simulink model "All_Controllers"  (R2019b)
settings: Solver=VariableStepAuto  StartTime=0.0  StopTime=100  RelTol=1e-3
values from neighbouring files (symbols this model uses):
  A = data(1:1500, 1:3)    [ANN4.m]
  bike_params = [g h b a lambda m]    [All_ControllersScript.m]
  FinalValue = 1    [All_ControllersScript.m]
  Init_Angle = 0    [All_ControllersScript.m]
  lambda = deg2rad(90-24)    [All_ControllersScript.m]
  Noise = 1    [All_ControllersScript.m]
  PathData = length(SimulinkPath)-1    [All_ControllersScript.m]
  sys_dicretePID = c2d(steer_sys, Tsm, 'matched')    [All_ControllersScript.m]
  Ts = 0.01    [All_ControllersScript.m]
  TsD = 0.1    [All_ControllersScript.m]
  Tsm = Ts/6    (= 0.00166666666667)    [All_ControllersScript.m]
  v = 14/3.6    (= 3.88888888889)    [All_ControllersScript.m]
undefined symbols (not defined in the file or in its folder): B, C, D
libraries: simulink x9, simulink_extras x5, dspsrcs4 x1, dspsigops x1
settings Model: Creator=npn13003  LastModifiedBy=hampu
settings DataIOCC: ReturnWorkspaceOutputs=off
settings DebuggingCC: ArithmeticOperatorsInVariantConditions=warning
settings SFSimCC: SimUseLocalCustomCode=off  CustomCodeUndefinedFunction=UseInterfaceOnly
settings RTWCC: RTWUseLocalCustomCode=off

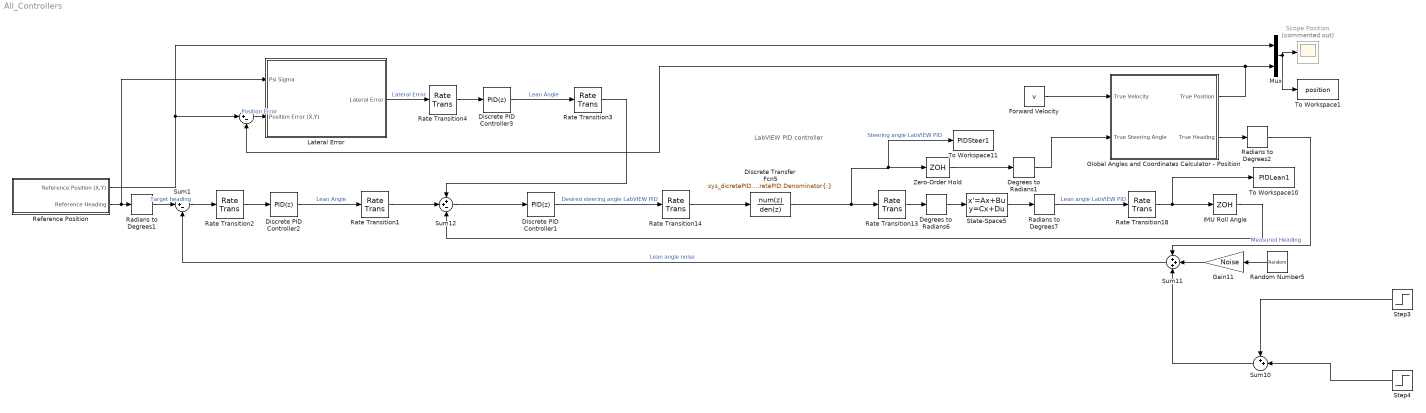
== system All_Controllers ==
  note: LabVIEW PID controller
  " " : Sum  Inputs=|+-
  Degrees to Radians1 : simulink_extras/Transformations/Degrees to Radians
  Degrees to Radians6 : simulink_extras/Transformations/Degrees to Radians
  Discrete Transfer Fcn5 : DiscreteTransferFcn  Numerator=sys_dicretePID.Numerator{:}  Denominator=sys_dicretePID.Denominator{:}
  Discrete PID Controller1 : simulink/Continuous/PID Controller  Controller=PID  Form=Ideal  TimeDomain=Discrete-time  SampleTime=Ts  IntegratorMethod=Trapezoidal  FilterMethod=Forward Euler  ControllerParametersSource=internal  P=3.418  I=1.327  D=0.0646  UseFilter=off  N=100  TunerSelectOption=Transfer Function Based (PID Tuner App)  InitialConditionSource=internal  InitialConditionForIntegrator=0  InitialConditionForFilter=0  DifferentiatorICPrevScaledInput=0  ExternalReset=none  TrackingMode=off  Kt=1  LimitOutput=off  UpperSaturationLimit=inf  LowerSaturationLimit=-inf  LinearizeAsGain=off  AntiWindupMode=none  Kb=1  POutMin=[]  POutMax=[]  IOutMin=[]  IOutMax=[]  DOutMin=[]  DOutMax=[]  NOutMin=[]  NOutMax=[]  SumOutMin=[]  SumOutMax=[]  SaturationOutMin=[]  SaturationOutMax=[]  PParamMin=[]  PParamMax=[]  IParamMin=[]  IParamMax=[]  DParamMin=[]  DParamMax=[]  NParamMin=[]  NParamMax=[]  KbParamMin=[]  KbParamMax=[]  KtParamMin=[]  KtParamMax=[]  KbOutMin=[]  KbOutMax=[]  KtOutMin=[]  KtOutMax=[]  IntegratorOutMin=[]  IntegratorOutMax=[]  FilterOutMin=[]  FilterOutMax=[]  SumI1OutMin=[]  SumI1OutMax=[]  SumI2OutMin=[]  SumI2OutMax=[]  SumI3OutMin=[]  SumI3OutMax=[]  SumI4OutMin=[]  SumI4OutMax=[]  SumDOutMin=[]  SumDOutMax=[]  DifferentiatorOutMin=[]  DifferentiatorOutMax=[]  FilterDiffOutCoefMin=[]  FilterDiffOutCoefMax=[]  ReciprocalOutMin=[]  ReciprocalOutMax=[]  SumDenOutMin=[]  SumDenOutMax=[]  SumNumOutMin=[]  SumNumOutMax=[]  DivideOutMin=[]  DivideOutMax=[]  IntegratorContinuousStateAttributes=''  IntegratorStateMustResolveToSignalObject=off  IntegratorRTWStateStorageClass=Auto  FilterContinuousStateAttributes=''  FilterStateMustResolveToSignalObject=off  FilterRTWStateStorageClass=Auto  ParallelPVariant=Passthrough  IdealPVariant=InternalParameters  IVariant=InternalParameters  DVariant=InternalParameters  IntegratorVariant=Discrete  SatVariant=Disabled  AWVariant=Passthrough  PCopyVariant=Disabled  TRVariant=Disabled  FdbkBlocksVariant=Forward  IdealPFdbkVariant=Disabled  SatFdbkVariant=Disabled  DerivativeFilterVariant=Differentiator  NVariant=Passthrough  NCopyVariant=Disabled_SignalSpec  FilterICVariant=InternalICsDifferentiator  IntegratorICVariant=InternalICs  ExternalResetVariant=Disabled  TRSumVariant=Passthrough  SumFdbkVariant=Disabled  SumVariant=Sum_PID
  Discrete PID Controller2 : simulink/Continuous/PID Controller  Controller=PID  Form=Ideal  TimeDomain=Discrete-time  SampleTime=TsD  IntegratorMethod=Trapezoidal  FilterMethod=Forward Euler  ControllerParametersSource=internal  P=-0.2  I=0  D=0  UseFilter=off  N=100  TunerSelectOption=Transfer Function Based (PID Tuner App)  InitialConditionSource=internal  InitialConditionForIntegrator=0  InitialConditionForFilter=0  DifferentiatorICPrevScaledInput=0  ExternalReset=none  TrackingMode=off  Kt=1  LimitOutput=off  UpperSaturationLimit=inf  LowerSaturationLimit=-inf  LinearizeAsGain=off  AntiWindupMode=none  Kb=1  POutMin=[]  POutMax=[]  IOutMin=[]  IOutMax=[]  DOutMin=[]  DOutMax=[]  NOutMin=[]  NOutMax=[]  SumOutMin=[]  SumOutMax=[]  SaturationOutMin=[]  SaturationOutMax=[]  PParamMin=[]  PParamMax=[]  IParamMin=[]  IParamMax=[]  DParamMin=[]  DParamMax=[]  NParamMin=[]  NParamMax=[]  KbParamMin=[]  KbParamMax=[]  KtParamMin=[]  KtParamMax=[]  KbOutMin=[]  KbOutMax=[]  KtOutMin=[]  KtOutMax=[]  IntegratorOutMin=[]  IntegratorOutMax=[]  FilterOutMin=[]  FilterOutMax=[]  SumI1OutMin=[]  SumI1OutMax=[]  SumI2OutMin=[]  SumI2OutMax=[]  SumI3OutMin=[]  SumI3OutMax=[]  SumI4OutMin=[]  SumI4OutMax=[]  SumDOutMin=[]  SumDOutMax=[]  DifferentiatorOutMin=[]  DifferentiatorOutMax=[]  FilterDiffOutCoefMin=[]  FilterDiffOutCoefMax=[]  ReciprocalOutMin=[]  ReciprocalOutMax=[]  SumDenOutMin=[]  SumDenOutMax=[]  SumNumOutMin=[]  SumNumOutMax=[]  DivideOutMin=[]  DivideOutMax=[]  IntegratorContinuousStateAttributes=''  IntegratorStateMustResolveToSignalObject=off  IntegratorRTWStateStorageClass=Auto  FilterContinuousStateAttributes=''  FilterStateMustResolveToSignalObject=off  FilterRTWStateStorageClass=Auto  ParallelPVariant=Passthrough  IdealPVariant=InternalParameters  IVariant=InternalParameters  DVariant=InternalParameters  IntegratorVariant=Discrete  SatVariant=Disabled  AWVariant=Passthrough  PCopyVariant=Disabled  TRVariant=Disabled  FdbkBlocksVariant=Forward  IdealPFdbkVariant=Disabled  SatFdbkVariant=Disabled  DerivativeFilterVariant=Differentiator  NVariant=Passthrough  NCopyVariant=Disabled_SignalSpec  FilterICVariant=InternalICsDifferentiator  IntegratorICVariant=InternalICs  ExternalResetVariant=Disabled  TRSumVariant=Passthrough  SumFdbkVariant=Disabled  SumVariant=Sum_PID
  Discrete PID Controller3 : simulink/Continuous/PID Controller  Controller=PID  Form=Ideal  TimeDomain=Discrete-time  SampleTime=TsD  IntegratorMethod=Trapezoidal  FilterMethod=Forward Euler  ControllerParametersSource=internal  P=-2  I=0  D=0  UseFilter=off  N=100  TunerSelectOption=Transfer Function Based (PID Tuner App)  InitialConditionSource=internal  InitialConditionForIntegrator=0  InitialConditionForFilter=0  DifferentiatorICPrevScaledInput=0  ExternalReset=none  TrackingMode=off  Kt=1  LimitOutput=off  UpperSaturationLimit=inf  LowerSaturationLimit=-inf  LinearizeAsGain=off  AntiWindupMode=none  Kb=1  POutMin=[]  POutMax=[]  IOutMin=[]  IOutMax=[]  DOutMin=[]  DOutMax=[]  NOutMin=[]  NOutMax=[]  SumOutMin=[]  SumOutMax=[]  SaturationOutMin=[]  SaturationOutMax=[]  PParamMin=[]  PParamMax=[]  IParamMin=[]  IParamMax=[]  DParamMin=[]  DParamMax=[]  NParamMin=[]  NParamMax=[]  KbParamMin=[]  KbParamMax=[]  KtParamMin=[]  KtParamMax=[]  KbOutMin=[]  KbOutMax=[]  KtOutMin=[]  KtOutMax=[]  IntegratorOutMin=[]  IntegratorOutMax=[]  FilterOutMin=[]  FilterOutMax=[]  SumI1OutMin=[]  SumI1OutMax=[]  SumI2OutMin=[]  SumI2OutMax=[]  SumI3OutMin=[]  SumI3OutMax=[]  SumI4OutMin=[]  SumI4OutMax=[]  SumDOutMin=[]  SumDOutMax=[]  DifferentiatorOutMin=[]  DifferentiatorOutMax=[]  FilterDiffOutCoefMin=[]  FilterDiffOutCoefMax=[]  ReciprocalOutMin=[]  ReciprocalOutMax=[]  SumDenOutMin=[]  SumDenOutMax=[]  SumNumOutMin=[]  SumNumOutMax=[]  DivideOutMin=[]  DivideOutMax=[]  IntegratorContinuousStateAttributes=''  IntegratorStateMustResolveToSignalObject=off  IntegratorRTWStateStorageClass=Auto  FilterContinuousStateAttributes=''  FilterStateMustResolveToSignalObject=off  FilterRTWStateStorageClass=Auto  ParallelPVariant=Passthrough  IdealPVariant=InternalParameters  IVariant=InternalParameters  DVariant=InternalParameters  IntegratorVariant=Discrete  SatVariant=Disabled  AWVariant=Passthrough  PCopyVariant=Disabled  TRVariant=Disabled  FdbkBlocksVariant=Forward  IdealPFdbkVariant=Disabled  SatFdbkVariant=Disabled  DerivativeFilterVariant=Differentiator  NVariant=Passthrough  NCopyVariant=Disabled_SignalSpec  FilterICVariant=InternalICsDifferentiator  IntegratorICVariant=InternalICs  ExternalResetVariant=Disabled  TRSumVariant=Passthrough  SumFdbkVariant=Disabled  SumVariant=Sum_PID
  Forward Velocity : Constant  Value=v
  Gain11 : Gain  Gain=Noise
  Global Angles and Coordinates Calculator - Position : Subsystem  SystemSampleTime=Ts
  IMU Roll Angle : ZeroOrderHold  SampleTime=Ts
  Lateral Error : Subsystem  SystemSampleTime=Ts
  Mux : Mux  Inputs=2
  Radians to Degrees1 : simulink_extras/Transformations/Radians to Degrees
  Radians to Degrees2 : simulink_extras/Transformations/Radians to Degrees
  Radians to Degrees7 : simulink_extras/Transformations/Radians to Degrees
  Random Number5 : RandomNumber  Variance=0.0001  SampleTime=Ts
  Rate Transition1 : RateTransition  OutPortSampleTime=Ts
  Rate Transition13 : RateTransition  OutPortSampleTime=0
  Rate Transition14 : RateTransition  OutPortSampleTime=Tsm
  Rate Transition18 : RateTransition  OutPortSampleTime=Ts
  Rate Transition2 : RateTransition  OutPortSampleTime=TsD
  Rate Transition3 : RateTransition  OutPortSampleTime=Ts
  Rate Transition4 : RateTransition  OutPortSampleTime=TsD
  Reference Position : Subsystem
  Scope Position : Scope  Commented=on
  State-Space5 : StateSpace  A=A  B=B  C=C  D=D  InitialCondition=[deg2rad(Init_Angle/C(1,1)) 0]
  Step3 : Step  Time=1.25  After=-FinalValue  SampleTime=Ts  VectorParams1D=off
  Step4 : Step  After=FinalValue  SampleTime=Ts  VectorParams1D=off
  Sum1 : Sum  Inputs=|+-
  Sum10 : Sum  Inputs=++|
  Sum11 : Sum  Inputs=+++
  Sum12 : Sum  Inputs=++-
  To Workspace1 : ToWorkspace  VariableName=position  SaveFormat=Timeseries  SampleTime=-1
  To Workspace10 : ToWorkspace  VariableName=PIDLean1  SampleTime=-1
  To Workspace11 : ToWorkspace  VariableName=PIDSteer1  SampleTime=-1
  Zero-Order Hold : ZeroOrderHold  SampleTime=Tsm
  wires:
  Step3/1 -> Sum10/1
  Step4/1 -> Sum10/2
  Rate Transition18/1 -> To Workspace10/1, IMU Roll Angle/1
  Degrees to Radians6/1 -> State-Space5/1
  Radians to Degrees7/1 -> Rate Transition18/1  "Lean angle LabVIEW PID"
  Rate Transition14/1 -> Discrete Transfer Fcn5/1
  Rate Transition13/1 -> Degrees to Radians6/1
  State-Space5/1 -> Radians to Degrees7/1
  Random Number5/1 -> Gain11/1
  Discrete Transfer Fcn5/1 -> Zero-Order Hold/1, To Workspace11/1, Rate Transition13/1  "Steering angle LabVIEW PID"
  Discrete PID Controller1/1 -> Rate Transition14/1  "Desired steering angle LabVIEW PID"
  Gain11/1 -> Sum11/2
  Sum10/1 -> Sum11/3
  Sum12/1 -> Discrete PID Controller1/1
  Discrete PID Controller2/1 -> Rate Transition1/1  "Lean Angle"
  Sum1/1 -> Rate Transition2/1
  Reference Position/2(Reference Heading) -> Lateral Error/1(Psi Sigma), Radians to Degrees1/1
  Rate Transition2/1 -> Discrete PID Controller2/1
  IMU Roll Angle/1 -> Sum12/3
  Mux/1 -> To Workspace1/1, Scope Position/1
  Zero-Order Hold/1 -> Degrees to Radians1/1
  Forward Velocity/1 -> Global Angles and Coordinates Calculator - Position/1(True Velocity)
  Degrees to Radians1/1 -> Global Angles and Coordinates Calculator - Position/2(True Steering Angle)
  Radians to Degrees1/1 -> Sum1/1  "Target heading"
  Global Angles and Coordinates Calculator - Position/2(True Heading) -> Radians to Degrees2/1
  Radians to Degrees2/1 -> Sum11/1  "Measured Heading"
  Rate Transition4/1 -> Discrete PID Controller3/1
  Rate Transition3/1 -> Sum12/1
  Discrete PID Controller3/1 -> Rate Transition3/1  "Lean Angle"
  Global Angles and Coordinates Calculator - Position/1(True Position) -> " "/2, Mux/2
  " "/1 -> Lateral Error/2(Position Error (X,Y))  "Position Error"
  Reference Position/1(Reference Position (X,Y)) -> Mux/1, " "/1
  Lateral Error/1(Lateral Error) -> Rate Transition4/1  "Lateral Error"
  Rate Transition1/1 -> Sum12/2
  Sum11/1 -> Sum1/2  "Lean angle noise"

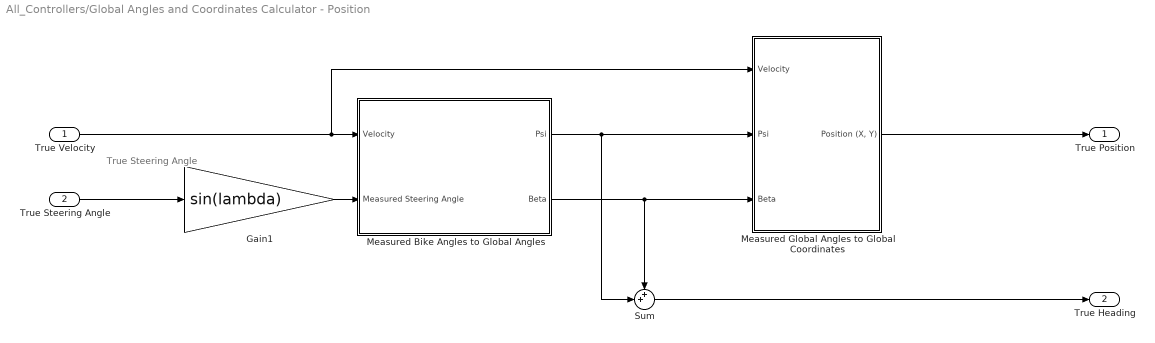
== system All_Controllers/Global Angles and Coordinates Calculator - Position ==
  note: True Steering
      | Angle
  True Velocity : Inport
  True Steering Angle : Inport  Port=2
  Gain1 : Gain  Gain=sin(lambda)
  Measured Bike Angles to Global Angles : Subsystem
  Measured Global Angles to Global Coordinates : Subsystem
  Sum : Sum  Inputs=++|
  True Position : Outport  VectorParamsAs1DForOutWhenUnconnected=off
  True Heading : Outport  Port=2  VectorParamsAs1DForOutWhenUnconnected=off
  wires:
  Measured Bike Angles to Global Angles/1(Psi) -> Sum/2, Measured Global Angles to Global Coordinates/2(Psi)
  Gain1/1 -> Measured Bike Angles to Global Angles/2(Measured Steering Angle)
  Sum/1 -> True Heading/1
  Measured Bike Angles to Global Angles/2(Beta) -> Sum/1, Measured Global Angles to Global Coordinates/3(Beta)
  Measured Global Angles to Global Coordinates/1("Position (X, Y)") -> True Position/1
  True Velocity/1 -> Measured Global Angles to Global Coordinates/1(Velocity), Measured Bike Angles to Global Angles/1(Velocity)
  True Steering Angle/1 -> Gain1/1

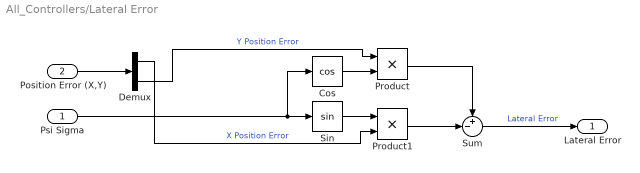
== system All_Controllers/Lateral Error ==
  Psi Sigma : Inport
  Position Error (X,Y) : Inport  Port=2
  Cos : Trigonometry  Operator=cos
  Demux : Demux  Outputs=2
  Product : Product
  Product1 : Product
  Sin : Trigonometry
  Sum : Sum  Inputs=+-|
  Lateral Error : Outport  VectorParamsAs1DForOutWhenUnconnected=off
  wires:
  Cos/1 -> Product/2
  Sin/1 -> Product1/1
  Psi Sigma/1 -> Cos/1, Sin/1
  Product1/1 -> Sum/2
  Product/1 -> Sum/1
  Sum/1 -> Lateral Error/1  "Lateral Error"
  Demux/1 -> Product1/2  "X Position Error"
  Demux/2 -> Product/1  "Y Position Error"
  Position Error (X,Y)/1 -> Demux/1

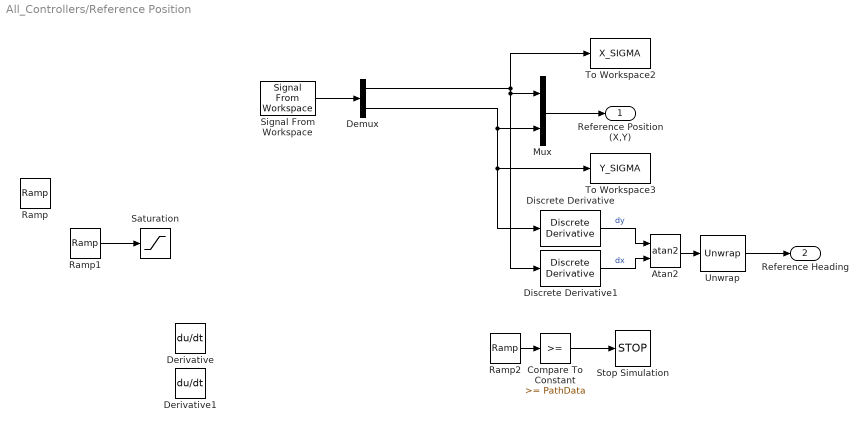
== system All_Controllers/Reference Position ==
  Atan2 : Trigonometry  Operator=atan2
  Compare To Constant : simulink/Logic and Bit Operations/Compare To Constant  relop=>=  const=PathData  OutDataTypeStr=boolean
  Demux : Demux  Outputs=2
  Derivative : Derivative
  Derivative1 : Derivative
  Discrete Derivative : simulink/Discrete/Discrete Derivative  gainval=1.0  ICPrevScaledInput=0.0  OutMin=[]  OutMax=[]  OutDataType=fixdt(1, 16)  OutScaling=2^-10  DoSatur=off
  Discrete Derivative1 : simulink/Discrete/Discrete Derivative  gainval=1.0  ICPrevScaledInput=0.0  OutMin=[]  OutMax=[]  OutDataType=fixdt(1, 16)  OutScaling=2^-10  DoSatur=off
  Mux : Mux  Inputs=2
  Ramp : simulink/Sources/Ramp  slope=3  start=0  InitialOutput=0
  Ramp1 : simulink/Sources/Ramp  slope=0.5  start=5  InitialOutput=0
  Ramp2 : simulink/Sources/Ramp  slope=1/TsD  start=0  InitialOutput=0
  Saturation : Saturate  UpperLimit=4  LowerLimit=0
  Signal From Workspace : dspsrcs4/Signal From Workspace  X=SimulinkPath  Ts=TsD  nsamps=1  OutputAfterFinalValue=Cyclic repetition  ignoreOrWarnInputAndFrameLengths=off  OutputFrames=off
  Stop Simulation : Stop
  To Workspace2 : ToWorkspace  VariableName=X_SIGMA  SaveFormat=Timeseries  SampleTime=TsD
  To Workspace3 : ToWorkspace  VariableName=Y_SIGMA  SaveFormat=Timeseries  SampleTime=TsD
  Unwrap : dspsigops/Unwrap  tol=pi  InputProcessing=Columns as channels (frame based)  running=off
  Reference Position (X,Y) : Outport  VectorParamsAs1DForOutWhenUnconnected=off
  Reference Heading : Outport  Port=2  VectorParamsAs1DForOutWhenUnconnected=off
  wires:
  Mux/1 -> Reference Position (X,Y)/1
  Demux/1 -> To Workspace2/1, Discrete Derivative1/1, Mux/1
  Discrete Derivative1/1 -> Atan2/2  "dx"
  Atan2/1 -> Unwrap/1
  Unwrap/1 -> Reference Heading/1
  Discrete Derivative/1 -> Atan2/1  "dy"
  Demux/2 -> Discrete Derivative/1, To Workspace3/1, Mux/2
  Ramp1/1 -> Saturation/1
  Signal From Workspace/1 -> Demux/1
  Ramp2/1 -> Compare To Constant/1
  Compare To Constant/1 -> Stop Simulation/1

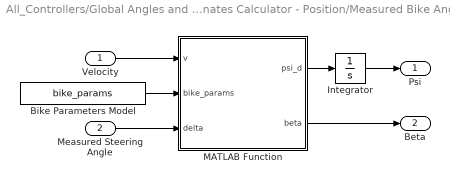
== system All_Controllers/Global Angles and Coordinates Calculator - Position/Measured Bike Angles to Global Angles ==
  Velocity : Inport
  Measured Steering Angle : Inport  Port=2
  " Bike Parameters Model " : Constant  Value=bike_params
  Integrator : Integrator
  MATLAB Function : MATLAB Function  TreatAsAtomicUnit=on
  Psi : Outport  VectorParamsAs1DForOutWhenUnconnected=off
  Beta : Outport  Port=2  VectorParamsAs1DForOutWhenUnconnected=off
  wires:
  MATLAB Function/2(beta) -> Beta/1
  MATLAB Function/1(psi_d) -> Integrator/1
  Integrator/1 -> Psi/1
  " Bike Parameters Model "/1 -> MATLAB Function/2(bike_params)
  Measured Steering Angle/1 -> MATLAB Function/3(delta)
  Velocity/1 -> MATLAB Function/1(v)

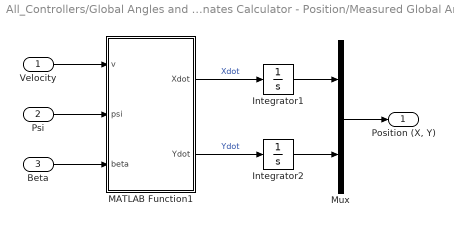
== system All_Controllers/Global Angles and Coordinates Calculator - Position/Measured Global Angles to Global Coordinates ==
  Velocity : Inport
  Psi : Inport  Port=2
  Beta : Inport  Port=3
  Integrator1 : Integrator
  Integrator2 : Integrator
  MATLAB Function1 : MATLAB Function  TreatAsAtomicUnit=on
  Mux : Mux  Inputs=2
  "Position (X, Y)" : Outport  VectorParamsAs1DForOutWhenUnconnected=off
  wires:
  MATLAB Function1/2(Ydot) -> Integrator2/1  "Ydot"
  MATLAB Function1/1(Xdot) -> Integrator1/1  "Xdot"
  Psi/1 -> MATLAB Function1/2(psi)
  Beta/1 -> MATLAB Function1/3(beta)
  Velocity/1 -> MATLAB Function1/1(v)
  Integrator2/1 -> Mux/2
  Integrator1/1 -> Mux/1
  Mux/1 -> "Position (X, Y)"/1

== matlab function All_Controllers/Global Angles and Coordinates Calculator - Position/Measured Bike Angles to Global Angles/MATLAB Function ==
  data: v input; bike_params input; delta input; psi_d output; beta output
function [psi_d, beta]  = fcn(v, bike_params, delta)

b = bike_params(3);
a = bike_params(4);

beta = atan((a / (b)) * tan(delta));
psi_d = (v / a) * sin(beta);

== matlab function All_Controllers/Global Angles and Coordinates Calculator - Position/Measured Global Angles to Global Coordinates/MATLAB Function1 ==
  data: v input; psi input; Xdot output; beta input; Ydot output
function [Xdot, Ydot]  = fcn(v, psi, beta)

Xdot = v * cos(psi + beta);
Ydot = v * sin(psi + beta);
